simulink model "control_JBT"  (R2021b)
settings: Solver=VariableStepAuto  StartTime=0.0  StopTime=10.0  RelTol=1e-3
settings Model: Creator=Pico  LastModifiedBy=Pico

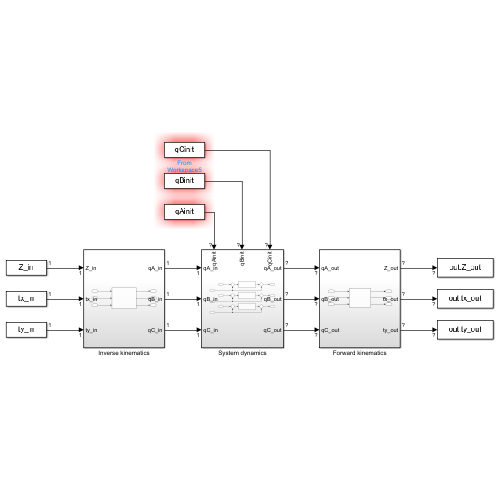
[thumbnail: Simulink's stored preview of the top-level diagram]
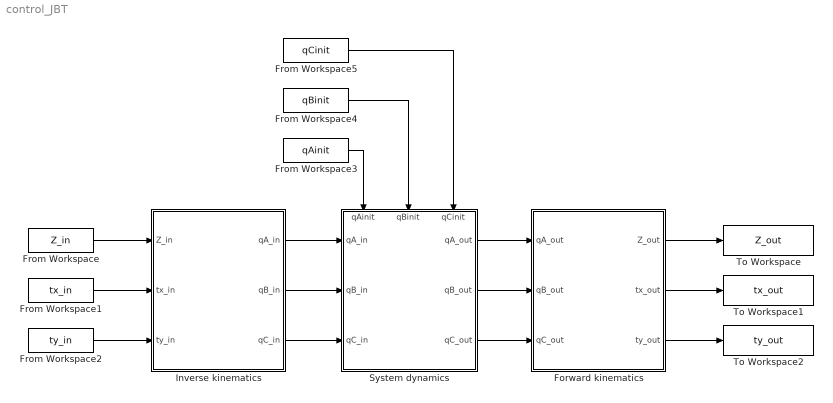
== system control_JBT ==
  Forward kinematics : Subsystem
  From Workspace : FromWorkspace  VariableName=Z_in  SampleTime=0.2
  From Workspace1 : FromWorkspace  VariableName=tx_in  SampleTime=0.2
  From Workspace2 : FromWorkspace  VariableName=ty_in  SampleTime=0.2
  From Workspace3 : FromWorkspace  VariableName=qAinit
  From Workspace4 : FromWorkspace  VariableName=qBinit
  From Workspace5 : FromWorkspace  VariableName=qCinit
  Inverse kinematics : Subsystem
  System dynamics : Subsystem
      settings: PortSchema="{\"entries\":[{\"content\":{\"sides\":[{\"content\":{\"connectorIds\":[\"In1\",\"In2\",\"In3\"]},\"type\":\"ConnectorPlacement.EquallySpacedRectSide\",\"uuid\":\"c24ee354-3a75-4f1b-83ec-264891b7fa65\"},{\"content\":{\"connectorIds\":[\"Out1\",\"Out2\",\"Out3\"],\"side\":\"RIGHT\"},\"type\":\"ConnectorPlacement.EquallySpacedRectSide\",\"uuid\":\"1c3c61c0-7ee5-4706-8614-71b4a13f5af9\"},{\"content\":{\"connectorIds\":[\"In4\",\"In5\",\"In6\"],\"side\":\"TOP\"},\"type\":\"ConnectorPlacement.EquallySpacedRectSide\",\"uuid\":\"e7485cef-0252-4699-ab67-c998e9ad588f\"}]},\"type\":\"ConnectorPlacement.EquallySpacedConnector\",\"uuid\":\"8b8049af-70f7-45f7-ad41-3dbd2e3f59b2\"}],\"packageUris\":[\"http://schema.mathworks.com/mf0/Connector/R2020b\"],\"version\":\"1.0\"}"
  To Workspace : ToWorkspace  VariableName=Z_out  SaveFormat=Timeseries  SampleTime=-1
  To Workspace1 : ToWorkspace  VariableName=tx_out  SaveFormat=Timeseries  SampleTime=-1
  To Workspace2 : ToWorkspace  VariableName=ty_out  SaveFormat=Timeseries  SampleTime=-1
  wires:
  From Workspace/1 -> Inverse kinematics/1(Z_in)
  From Workspace1/1 -> Inverse kinematics/2(tx_in)
  From Workspace2/1 -> Inverse kinematics/3(ty_in)
  Inverse kinematics/1(qA_in) -> System dynamics/1(qA_in)
  Inverse kinematics/2(qB_in) -> System dynamics/2(qB_in)
  Inverse kinematics/3(qC_in) -> System dynamics/3(qC_in)
  System dynamics/1(qA_out) -> Forward kinematics/1(qA_out)
  System dynamics/2(qB_out) -> Forward kinematics/2(qB_out)
  System dynamics/3(qC_out) -> Forward kinematics/3(qC_out)
  Forward kinematics/1(Z_out) -> To Workspace/1
  Forward kinematics/2(tx_out) -> To Workspace1/1
  Forward kinematics/3(ty_out) -> To Workspace2/1
  From Workspace3/1 -> System dynamics/4(qAinit)
  From Workspace4/1 -> System dynamics/5(qBinit)
  From Workspace5/1 -> System dynamics/6(qCinit)

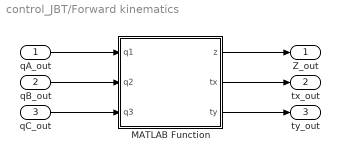
== system control_JBT/Forward kinematics ==
  qA_out : Inport
  qB_out : Inport  Port=2
  qC_out : Inport  Port=3
  MATLAB Function : MATLAB Function  TreatAsAtomicUnit=on
  Z_out : Outport
  tx_out : Outport  Port=2
  ty_out : Outport  Port=3
  wires:
  qA_out/1 -> MATLAB Function/1(q1)
  MATLAB Function/1(z) -> Z_out/1
  qB_out/1 -> MATLAB Function/2(q2)
  MATLAB Function/2(tx) -> tx_out/1
  qC_out/1 -> MATLAB Function/3(q3)
  MATLAB Function/3(ty) -> ty_out/1

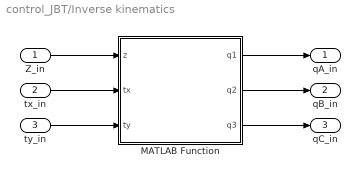
== system control_JBT/Inverse kinematics ==
  Z_in : Inport
  tx_in : Inport  Port=2
  ty_in : Inport  Port=3
  MATLAB Function : MATLAB Function  TreatAsAtomicUnit=on
  qA_in : Outport
  qB_in : Outport  Port=2
  qC_in : Outport  Port=3
  wires:
  Z_in/1 -> MATLAB Function/1(z)
  MATLAB Function/1(q1) -> qA_in/1
  tx_in/1 -> MATLAB Function/2(tx)
  MATLAB Function/2(q2) -> qB_in/1
  ty_in/1 -> MATLAB Function/3(ty)
  MATLAB Function/3(q3) -> qC_in/1

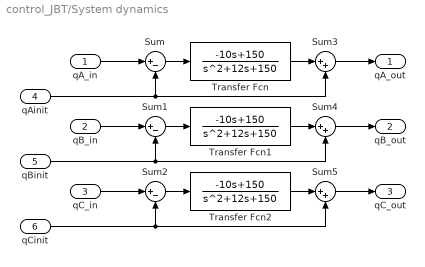
== system control_JBT/System dynamics ==
  qA_in : Inport
  qB_in : Inport  Port=2
  qC_in : Inport  Port=3
  qAinit : Inport  Port=4
  qBinit : Inport  Port=5
  qCinit : Inport  Port=6
  Sum : Sum  Inputs=|+-
  Sum1 : Sum  Inputs=|+-
  Sum2 : Sum  Inputs=|+-
  Sum3 : Sum  Inputs=|++
  Sum4 : Sum  Inputs=|++
  Sum5 : Sum  Inputs=|++
  Transfer Fcn : TransferFcn  Numerator=[-10 150]  Denominator=[1 12 150]
  Transfer Fcn1 : TransferFcn  Numerator=[-10 150]  Denominator=[1 12 150]
  Transfer Fcn2 : TransferFcn  Numerator=[-10 150]  Denominator=[1 12 150]
  qA_out : Outport
  qB_out : Outport  Port=2
  qC_out : Outport  Port=3
  wires:
  qA_in/1 -> Sum/1
  Sum/1 -> Transfer Fcn/1
  Transfer Fcn/1 -> Sum3/1
  Sum4/1 -> qB_out/1
  qB_in/1 -> Sum1/1
  qC_in/1 -> Sum2/1
  Sum3/1 -> qA_out/1
  Sum5/1 -> qC_out/1
  qBinit/1 -> Sum4/2, Sum1/2
  Sum1/1 -> Transfer Fcn1/1
  Transfer Fcn1/1 -> Sum4/1
  Sum2/1 -> Transfer Fcn2/1
  Transfer Fcn2/1 -> Sum5/1
  qAinit/1 -> Sum/2, Sum3/2
  qCinit/1 -> Sum5/2, Sum2/2

== matlab function control_JBT/Forward kinematics/MATLAB Function ==
  data: q1 input; z output; q2 input; q3 input; tx output; ty output
function [z, tx, ty] = fwd_kin(q1, q2, q3)
%%
% This function computes the inverse kinematics of the bouncing table given
% the desired end effector height (z), and the angles (tx and ty) that the
% end effector makes with the x and y axes, respectively. It uses a lookup
% table of precomputed joint angles (qA, qB, and qC) and corresponding
% end effector positions (Z, theta_x, and theta_y) to find the joint angles
% that produce the desired end effector position.
%
% Inputs:
% z - Scalar value representing the desired height of the end effector.
% tx - Scalar value representing the desired angle that the end effector makes with the x-axis.
% ty - Scalar value representing the desired angle that the end effector makes with the y-axis.
% lookup_table - A structure containing the precomputed joint angles 
% (qA, qB, and qC) and corresponding end effector positions 
% (Z, theta_x, and theta_y).
%
% Outputs:
% q1 - the closest joint angle qA that produces the desired end effector position.
% q2 - the closest joint angle qB that produces the desired end effector position.
% q3 - the closest joint angle qC that produces the desired end effector position.
%
%%
lookup_table = load('lookup_table_v1_dq1.mat');
% Extracting the relevant data from the lookup table
Z = lookup_table.Z;
theta_x = lookup_table.theta_x;
theta_y = lookup_table.theta_y;
qA = lookup_table.qA;
qB = lookup_table.qB;
qC = lookup_table.qC;

% Computing the Euclidean distance between the desired position and all entries in the table
dist = sqrt((qA(:) - q1).^2 + (qB(:) - q2).^2 + (qC(:) - q3).^2);

% Finding the index of the entry with the smallest distance
[~, index] = min(dist);

% Getting the corresponding joint angles
z = Z(index);
tx = theta_x(index);
ty = theta_y(index);

end

== matlab function control_JBT/Inverse kinematics/MATLAB Function ==
  data: z input; q1 output; tx input; ty input; q2 output; q3 output
function [q1, q2, q3] = inv_kin(z, tx, ty)
%%
% This function computes the inverse kinematics of the bouncing table given
% the desired end effector height (z), and the angles (tx and ty) that the
% end effector makes with the x and y axes, respectively. It uses a lookup
% table of precomputed joint angles (qA, qB, and qC) and corresponding
% end effector positions (Z, theta_x, and theta_y) to find the joint angles
% that produce the desired end effector position.
%
% Inputs:
% z - Scalar value representing the desired height of the end effector.
% tx - Scalar value representing the desired angle that the end effector makes with the x-axis.
% ty - Scalar value representing the desired angle that the end effector makes with the y-axis.
% lookup_table - A structure containing the precomputed joint angles 
% (qA, qB, and qC) and corresponding end effector positions 
% (Z, theta_x, and theta_y).
%
% Outputs:
% q1 - the closest joint angle qA that produces the desired end effector position.
% q2 - the closest joint angle qB that produces the desired end effector position.
% q3 - the closest joint angle qC that produces the desired end effector position.
%
%%
lookup_table = load('lookup_table_v1_dq1.mat');
% Extracting the relevant data from the lookup table
Z = lookup_table.Z;
theta_x = lookup_table.theta_x;
theta_y = lookup_table.theta_y;
qA = lookup_table.qA;
qB = lookup_table.qB;
qC = lookup_table.qC;

% Computing the Euclidean distance between the desired position and all entries in the table
dist = sqrt((Z(:) - z).^2 + (theta_x(:) - tx).^2 + (theta_y(:) - ty).^2);

% Finding the index of the entry with the smallest distance
[~, index] = min(dist);

% Getting the corresponding joint angles
q1 = qA(index);
q2 = qB(index);
q3 = qC(index);

end
